simulink model "automotive_system"  (R2020b)
settings: Solver=ode23  StartTime=0.0  StopTime=50  MaxStep=0.0001  RelTol=1e-3
values from neighbouring files (symbols this model uses):
  b1 = 350    [constant_declaration.m]
  b2 = 15020    [constant_declaration.m]
  k1 = 80000    [constant_declaration.m]
  k2 = 500000    [constant_declaration.m]
  Kd = 208025    [constant_declaration.m]
  Ki = 624075    [constant_declaration.m]
  Kp = 832100    [constant_declaration.m]
  m1 = 2500    [constant_declaration.m]
  m2 = 320    [constant_declaration.m]
undefined symbols (not defined in the file or in its folder): sigbuilder_block
libraries: simulink x1
settings Model: Creator=shraddha  LastModifiedBy=shraddha

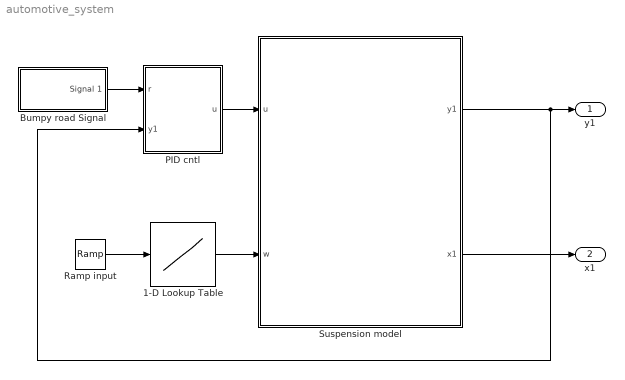
== system automotive_system ==
  1-D Lookup Table : Lookup_n-D  NumberOfTableDimensions=1  BreakpointsForDimension1=[0 1]  Table=[0 2]  InternalRulePriority=Speed  RndMeth=Simplest  InputSameDT=on
  "Bumpy road Signal " : Subsystem  Tag=STV Subsys  LoadFcn=sigbuilder_block('load');  StartFcn=sigbuilder_block('start');  StopFcn=sigbuilder_block('stop');  ClipboardFcn=sigbuilder_block('clipboard');  mask(Sigbuilder block){tuvar=[0:10]}
      mask help: Simulink:masks:SigbuilderBlock_MD
      mask init:
      | if ~strcmp(get_param(bdroot(gcbh),'SimulationStatus'),'stopped') tuvar = sigbuilder_block('maskInit'); end
      settings: CopyFcn=sigbuilder_block('copy');  DeleteFcn=sigbuilder_block('delete');  ModelCloseFcn=sigbuilder_block('modelClose');  PreSaveFcn=sigbuilder_block('preSave');  PauseFcn=sigbuilder_block('pause');  ContinueFcn=sigbuilder_block('continue');  NameChangeFcn=sigbuilder_block('namechange');  OpenFcn=sigbuilder_block('open',[437.6 153 550.4 359.25 ]);  CloseFcn=sigbuilder_block('close');
      mask Display: plot(0, 0, 100, 100,[2, 2, 32, 32, 2], [68, 8, 8, 68, 68],[32, 2], [38, 38], [32, 19, 2],[53, 60, 44], [32, 17, 17, 2],[16, 16, 31, 31]);txt = getActiveGroup(gcbh);text(2, 100, txt,'verticalAlignment', 'top');
  PID cntl : Subsystem
  Ramp input : simulink/Sources/Ramp  slope=1  start=0  InitialOutput=0
  Suspension model : Subsystem  InitFcn=|
      | m1 = 2500;
      | m2 = 320;
      | k1 = 80000;
      | k2 = 500000;
      | b1 = 350;
      | b2 = 15020;
      | Kd = 208025;
      | Kp = 832100;
      | Ki = 624075;
  y1 : Outport
  x1 : Outport  Port=2
  wires:
  "Bumpy road Signal "/1(Signal 1) -> PID cntl/1(r)
  Suspension model/1(y1) -> PID cntl/2(y1), y1/1
  PID cntl/1(u) -> Suspension model/1(u)
  Ramp input/1 -> 1-D Lookup Table/1
  1-D Lookup Table/1 -> Suspension model/2(w)
  Suspension model/2(x1) -> x1/1

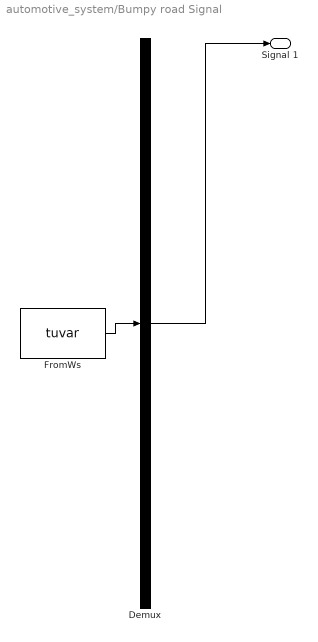
== system automotive_system/Bumpy road Signal  ==
  Demux : Demux  Tag=STV Demux  Outputs=1
      settings: DisplayOption=none
  FromWs : FromWorkspace  Tag=STV FromWs  VariableName=tuvar
      SigBuilderData=|
      | common.afterFinalStr = 'Extrapolate'
      | common.sampleTime = 0
      | dataSet.timeRange = [0 50]
      | dataSet.name = 'Group 1'
      | sbobj.Groups.Name = 'Group 1'
      | sbobj.Groups.Signals.Name = 'Signal 1'
      | sbobj.Groups.Signals.XData = [0 10 10 30 30 50]
      | sbobj.Groups.Signals.YData = [0 0 1 1 0 0]
      | sbobj.Groups.TimeRange = [0 50]
  Signal 1 : Outport  Tag=STV Outport
  wires:
  Demux/1 -> Signal 1/1
  FromWs/1 -> Demux/1

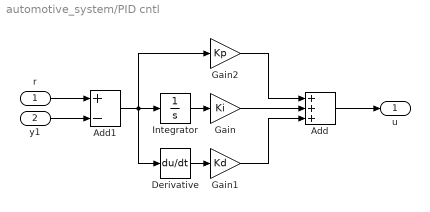
== system automotive_system/PID cntl ==
  r : Inport
  y1 : Inport  Port=2
  Add : Sum  Inputs=+++
  Add1 : Sum  Inputs=+-
  Derivative : Derivative
  Gain : Gain  Gain=Ki
  Gain1 : Gain  Gain=Kd
  Gain2 : Gain  Gain=Kp
  Integrator : Integrator
  u : Outport
  wires:
  Gain1/1 -> Add/3
  Add1/1 -> Integrator/1, Gain2/1, Derivative/1
  Gain/1 -> Add/2
  Integrator/1 -> Gain/1
  y1/1 -> Add1/2
  Gain2/1 -> Add/1
  Derivative/1 -> Gain1/1
  r/1 -> Add1/1
  Add/1 -> u/1

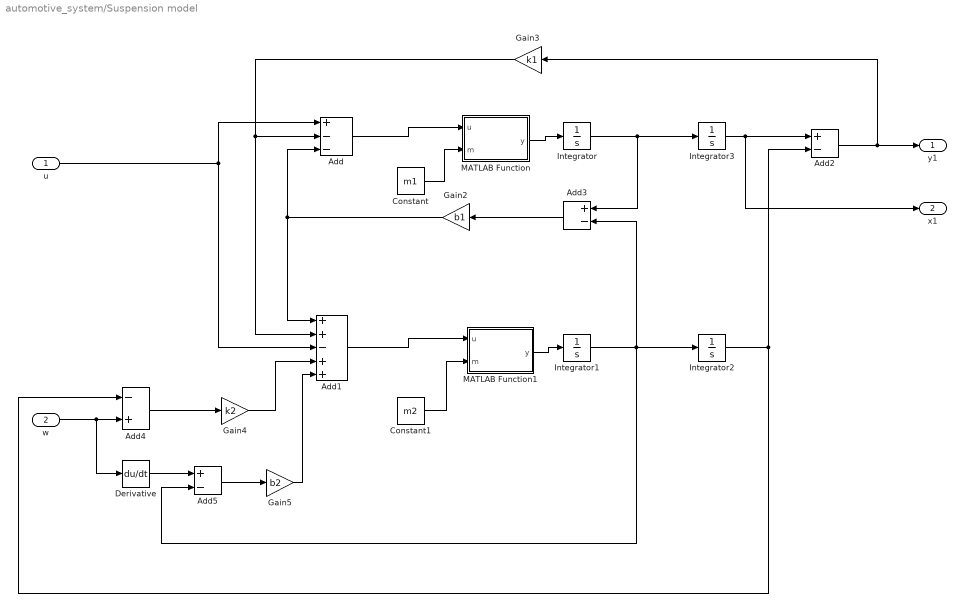
== system automotive_system/Suspension model ==
  u : Inport
  w : Inport  Port=2
  Add : Sum  Inputs=+--
  Add1 : Sum  Inputs=++-++
  Add2 : Sum  Inputs=+-
  Add3 : Sum  Inputs=+-
  Add4 : Sum  Inputs=-+
  Add5 : Sum  Inputs=+-
  Constant : Constant  Value=m1
  Constant1 : Constant  Value=m2
  Derivative : Derivative
  Gain2 : Gain  Gain=b1
  Gain3 : Gain  Gain=k1
  Gain4 : Gain  Gain=k2
  Gain5 : Gain  Gain=b2
  Integrator{,1..3} (4 alike) : Integrator
  MATLAB Function : MATLAB Function  TreatAsAtomicUnit=on
  MATLAB Function1 : MATLAB Function  TreatAsAtomicUnit=on
  y1 : Outport
  x1 : Outport  Port=2
  wires:
  Integrator1/1 -> Add5/2, Add3/2, Integrator2/1
  u/1 -> Add1/3, Add/1
  Integrator2/1 -> Add2/2, Add4/1
  w/1 -> Add4/2, Derivative/1
  Add2/1 -> y1/1, Gain3/1
  Integrator/1 -> Add3/1, Integrator3/1
  Add/1 -> MATLAB Function/1(u)
  Add3/1 -> Gain2/1
  Integrator3/1 -> x1/1, Add2/1
  Add5/1 -> Gain5/1
  Derivative/1 -> Add5/1
  Add4/1 -> Gain4/1
  Gain5/1 -> Add1/5
  Gain3/1 -> Add1/2, Add/2
  Add1/1 -> MATLAB Function1/1(u)
  Gain2/1 -> Add1/1, Add/3
  Gain4/1 -> Add1/4
  MATLAB Function/1(y) -> Integrator/1
  MATLAB Function1/1(y) -> Integrator1/1
  Constant/1 -> MATLAB Function/2(m)
  Constant1/1 -> MATLAB Function1/2(m)

== matlab function automotive_system/Suspension model/MATLAB Function ==
  data: u input; y output; m input
function y = fcn(u, m)

y = u/m;
end

== matlab function automotive_system/Suspension model/MATLAB Function1 ==
  data: u input; y output; m input
function y = fcn(u,m)

y = u/m;
